simulink model "ARPOD"  (R2019b)
settings: Solver=VariableStepAuto  StartTime=0.0  StopTime=240  RelTol=1e-3
model workspace (MAT data in the model file):
  x0_mode2 = Simulink.Parameter
  x0_mode2.DataType = 'auto'
  x0_mode2.Dimensions = [0 0]
values from neighbouring files (symbols this model uses):
  G11 = 3*n^2 -Glqr(1,1)/m    [init.m]
  G12 = -Glqr(1,2)/m    [init.m]
  G13 = -Glqr(1,3)/m    [init.m]
  G14 = 2*n -Glqr(1,4)/m    [init.m]
  G21 = -Glqr(2,1)/m    [init.m]
  G22 = -Glqr(2,2)/m    [init.m]
  G23 = -2*n -Glqr(2,3)/m    [init.m]
  G24 = -Glqr(2,4)/m    [init.m]
  K11 = 3*n^2 -Klqr(1,1)/m    [init.m]
  K12 = -Klqr(1,2)/m    [init.m]
  K13 = -Klqr(1,3)/m    [init.m]
  K14 = 2*n -Klqr(1,4)/m    [init.m]
  K21 = -Klqr(2,1)/m    [init.m]
  K22 = -Klqr(2,2)/m    [init.m]
  K23 = -2*n -Klqr(2,3)/m    [init.m]
  K24 = -Klqr(2,4)/m    [init.m]
undefined symbols (not defined in the file or in its folder): vx0, vx0_mode2, vy0, vy0_mode2, x0, y0, y0_mode2
libraries: simulink x1
settings Model: Creator=yuxia  LastModifiedBy=yuxia

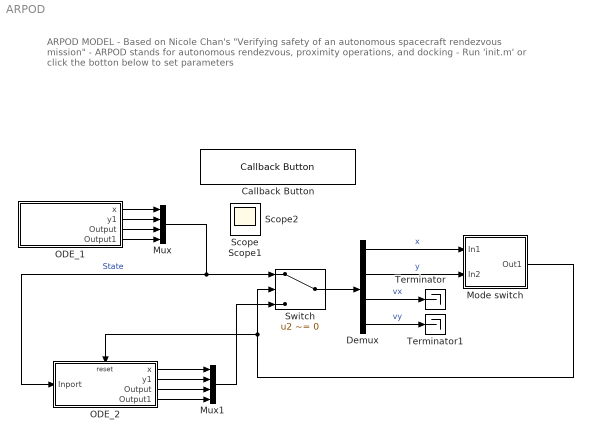
== system ARPOD ==
  note: ARPOD MODEL
      |
      | - Based on Nicole Chan's "Verifying safety of an autonomous spacecraft rendezvous mission"
      | - ARPOD stands for autonomous rendezvous, proximity operations, and docking
      | - Run 'init.m' or click the botton below to set parameters
  Callback Button : CallbackButton  ButtonText=CLICK TO INITIALIZE
      settings: ClickFcn=run 'init.m'
  Demux : Demux
  Mode switch : Subsystem
  Mux : Mux
  Mux1 : Mux
  ODE_1 : Subsystem
  ODE_2 : Subsystem
  Switch : Switch  Criteria=u2 ~= 0  Threshold=1
  Terminator : Terminator
  Terminator1 : Terminator
  Scope : Scope
  Scope1 : Scope
  Scope2 : Scope
  wires:
  ODE_1/1(x) -> Mux/1
  ODE_1/2(y1) -> Mux/2
  Switch/1 -> Demux/1
  ODE_2/1(x) -> Mux1/1
  ODE_2/2(y1) -> Mux1/2
  ODE_1/3(Output) -> Mux/3
  ODE_1/4(Output1) -> Mux/4
  ODE_2/3(Output) -> Mux1/3
  ODE_2/4(Output1) -> Mux1/4
  Mux/1 -> Switch/1, ODE_2/1(Inport)  "State"
  Mode switch/1(Out1) -> Switch/2, ODE_2/Reset
  Demux/3 -> Terminator/1  "vx"
  Demux/4 -> Terminator1/1  "vy"
  Demux/1 -> Mode switch/1(In1)  "x"
  Demux/2 -> Mode switch/2(In2)  "y"
  Mux1/1 -> Switch/3

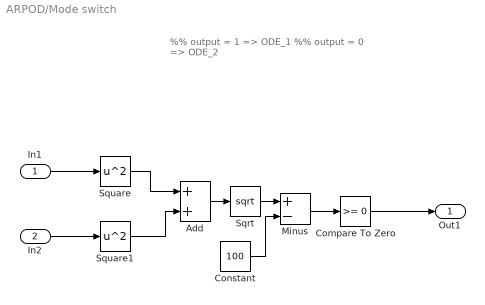
== system ARPOD/Mode switch ==
  note: %% output = 1 => ODE_1
      | %% output = 0 => ODE_2
  In1 : Inport
  In2 : Inport  Port=2
  Add : Sum
  Compare To Zero : simulink/Logic and Bit Operations/Compare To Zero  relop=>=  OutDataTypeStr=boolean
  Constant : Constant  Value=100
  Minus : Sum  Inputs=+-
  Sqrt : Sqrt  SaturateOnIntegerOverflow=on
  Square : Math  Operator=square  SignedPower=off  SaturateOnIntegerOverflow=on
  Square1 : Math  Operator=square  SignedPower=off  SaturateOnIntegerOverflow=on
  Out1 : Outport
  wires:
  Square/1 -> Add/1
  Square1/1 -> Add/2
  Constant/1 -> Minus/2
  Minus/1 -> Compare To Zero/1
  Compare To Zero/1 -> Out1/1
  Sqrt/1 -> Minus/1
  Add/1 -> Sqrt/1
  In1/1 -> Square/1
  In2/1 -> Square1/1

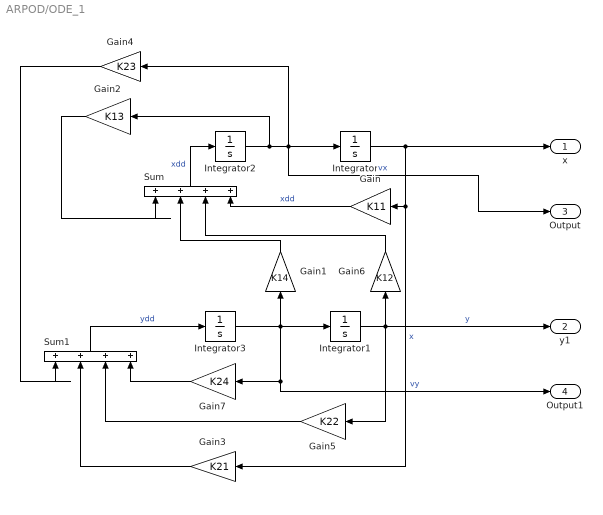
== system ARPOD/ODE_1 ==
  Gain : Gain  Gain=K11
  Gain1 : Gain  Gain=K14
  Gain2 : Gain  Gain=K13
  Gain3 : Gain  Gain=K21
  Gain4 : Gain  Gain=K23
  Gain5 : Gain  Gain=K22
  Gain6 : Gain  Gain=K12
  Gain7 : Gain  Gain=K24
  Integrator : Integrator  InitialCondition=x0
  Integrator1 : Integrator  InitialCondition=y0
  Integrator2 : Integrator  InitialCondition=vx0
  Integrator3 : Integrator  InitialCondition=vy0
  Sum : Sum  Inputs=|++++
  Sum1 : Sum  Inputs=|++++
  x : Outport
  y1 : Outport  Port=2
  Output : Outport  Port=3
  Output1 : Outport  Port=4
  wires:
  Gain1/1 -> Sum/2
  Gain5/1 -> Sum1/3
  Gain2/1 -> Sum/1
  Sum1/1 -> Integrator3/1  "ydd"
  Gain7/1 -> Sum1/4
  Gain3/1 -> Sum1/2
  Gain6/1 -> Sum/3
  Gain4/1 -> Sum1/1
  Integrator1/1 -> y1/1, Gain5/1, Gain6/1  "y"
  Integrator/1 -> x/1, Gain3/1, Gain/1  "x"
  Integrator2/1 -> Output/1, Gain4/1, Integrator/1, Gain2/1  "vx"
  Integrator3/1 -> Output1/1, Gain7/1, Integrator1/1, Gain1/1  "vy"
  Gain/1 -> Sum/4  "xdd"
  Sum/1 -> Integrator2/1  "xdd"

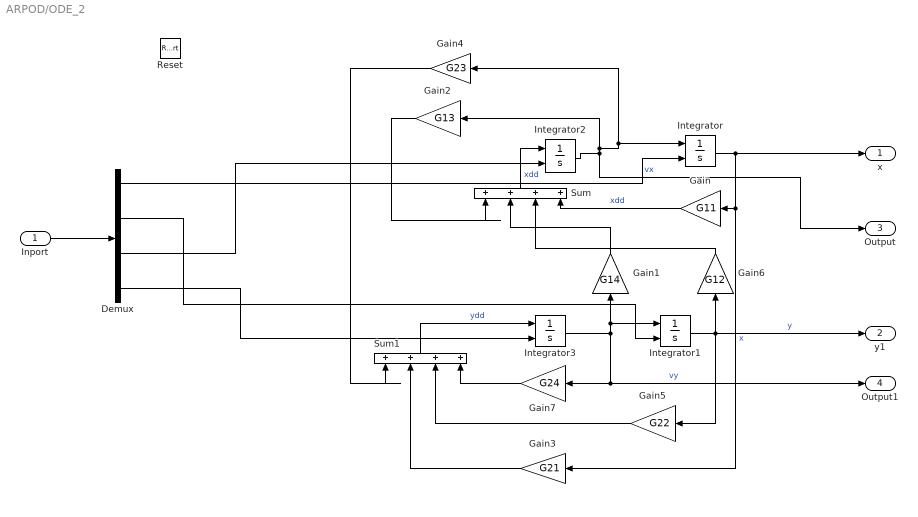
== system ARPOD/ODE_2 ==
  Inport : Inport
  Reset : ResetPort  DisableCoverage=on
  Demux : Demux
  Gain : Gain  Gain=G11
  Gain1 : Gain  Gain=G14
  Gain2 : Gain  Gain=G13
  Gain3 : Gain  Gain=G21
  Gain4 : Gain  Gain=G23
  Gain5 : Gain  Gain=G22
  Gain6 : Gain  Gain=G12
  Gain7 : Gain  Gain=G24
  Integrator : Integrator  InitialConditionSource=external  InitialCondition=x0_mode2
  Integrator1 : Integrator  InitialConditionSource=external  InitialCondition=y0_mode2
  Integrator2 : Integrator  InitialConditionSource=external  InitialCondition=vx0_mode2
  Integrator3 : Integrator  InitialConditionSource=external  InitialCondition=vy0_mode2
  Sum : Sum  Inputs=|++++
  Sum1 : Sum  Inputs=|++++
  x : Outport
  y1 : Outport  Port=2
  Output : Outport  Port=3
  Output1 : Outport  Port=4
  wires:
  Gain6/1 -> Sum/3
  Gain2/1 -> Sum/1
  Gain5/1 -> Sum1/3
  Gain/1 -> Sum/4  "xdd"
  Gain7/1 -> Sum1/4
  Gain3/1 -> Sum1/2
  Gain4/1 -> Sum1/1
  Sum/1 -> Integrator2/1  "xdd"
  Integrator/1 -> x/1, Gain3/1, Gain/1  "x"
  Sum1/1 -> Integrator3/1  "ydd"
  Integrator2/1 -> Gain4/1, Integrator/1, Gain2/1, Output/1  "vx"
  Integrator3/1 -> Integrator1/1, Gain1/1, Output1/1, Gain7/1  "vy"
  Gain1/1 -> Sum/2
  Integrator1/1 -> Gain6/1, y1/1, Gain5/1  "y"
  Inport/1 -> Demux/1
  Demux/1 -> Integrator/2
  Demux/2 -> Integrator1/2
  Demux/3 -> Integrator2/2
  Demux/4 -> Integrator3/2
